simulink model "QuarterCar_TS"  (R2014a)
settings: Solver=ode4  StartTime=0.0  StopTime=5  FixedStep=0.001  RelTol=1e-3
settings Model: Creator=MLRida  LastModifiedBy=MLRida

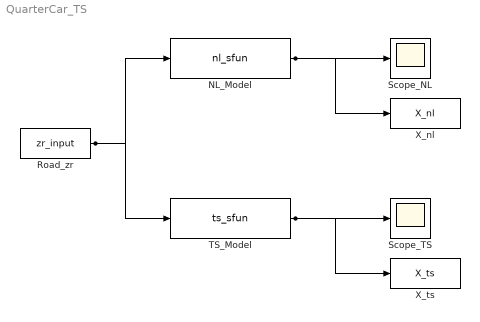
== system QuarterCar_TS ==
  NL_Model : S-Function  FunctionName=nl_sfun  EnableBusSupport=off
  Road_zr : FromWorkspace  VariableName=zr_input  SampleTime=0.001
  Scope_NL : Scope
  Scope_TS : Scope
  TS_Model : S-Function  FunctionName=ts_sfun  EnableBusSupport=off
  X_nl : ToWorkspace  VariableName=X_nl  SampleTime=-1
  X_ts : ToWorkspace  VariableName=X_ts  SampleTime=-1
  wires:
  Road_zr/1 -> NL_Model/1, TS_Model/1
  NL_Model/1 -> Scope_NL/1, X_nl/1
  TS_Model/1 -> Scope_TS/1, X_ts/1
